simulink model "PV_Copy_of_Flight_controller_LQR_r2019a"  (R2019a)
settings: Solver=FixedStepDiscrete  StartTime=0.0  StopTime=10.0  FixedStep=sample_time  RelTol=1e-3
PreLoadFcn:
  | init_s
InitFcn:
  | init_s
undefined symbols (not defined in the file or in its folder): fw_params_fc, G, K, k1_nlin, k2_nlin, k3_nlin, mixer, sample_time
Description:
  | Template for Flight_controller.
  | This model should be used as a basis to develop a custom controller.
  | The controller can be deployed to the drone by means of the
  | ANT-X SLXtoPX4 tool for automatic controller code generation.
settings Model: Creator=flyart  LastModifiedBy=mariam
settings DataIOCC: ReturnWorkspaceOutputs=off
settings OptimizationCC: BlockReduction=off  DefaultParameterBehavior=Inlined  DefaultUnderspecifiedDataType=single  InlineInvariantSignals=on  EnhancedBackFolding=on  CachingGlobalReferences=on  LocalBlockOutputs=off
settings DebuggingCC: ParameterTunabilityLossMsg=error  ArithmeticOperatorsInVariantConditions=warning
settings HardwareCC: ProdBitPerPointer=32  ProdBitPerSizeT=32  ProdBitPerPtrDiffT=32  ProdLargestAtomicInteger=Long  ProdLargestAtomicFloat=Double  ProdWordSize=32  ProdHWDeviceType=ARM Compatible->ARM Cortex
settings SFSimCC: SimUseLocalCustomCode=off  MATLABDynamicMemAlloc=off
settings RTWCC: SystemTargetFile=ert.tlc  GenCodeOnly=on  TemplateMakefile=ert_default_tmf  GenerateReport=on  RTWUseLocalCustomCode=off  Toolchain=GNU gcc/g++ | gmake (64-bit Linux)  BuildConfiguration=Faster Runs  IncludeHyperlinkInReport=on  LaunchReport=on  TargetLang=C++  GenerateTraceInfo=on  GenerateTraceReport=on  GenerateTraceReportSl=on  GenerateTraceReportSf=on  GenerateTraceReportEml=on  GenerateCodeMetricsReport=on
settings CodeAppCC: ForceParamTrailComments=on  OperatorAnnotations=on  SimulinkDataObjDesc=on  SFDataObjDesc=on  MATLABFcnDesc=on  CustomSymbolStrGlobalVar=rt$N$M  CustomSymbolStrType=$N$M  InsertBlockDesc=on  StateflowObjectComments=on  MATLABSourceComments=on
settings ERTTargetCC: MultiwordLength=2048  MultiInstanceERTCode=on  CodeInterfacePackaging=C++ class  SupportNonFinite=off  SupportComplex=off  InlinedParameterPlacement=NonHierarchical  RootIOFormat=Structure reference  ERTCustomFileTemplate=example_file_process.tlc  ERTFilePackagingFormat=Compact

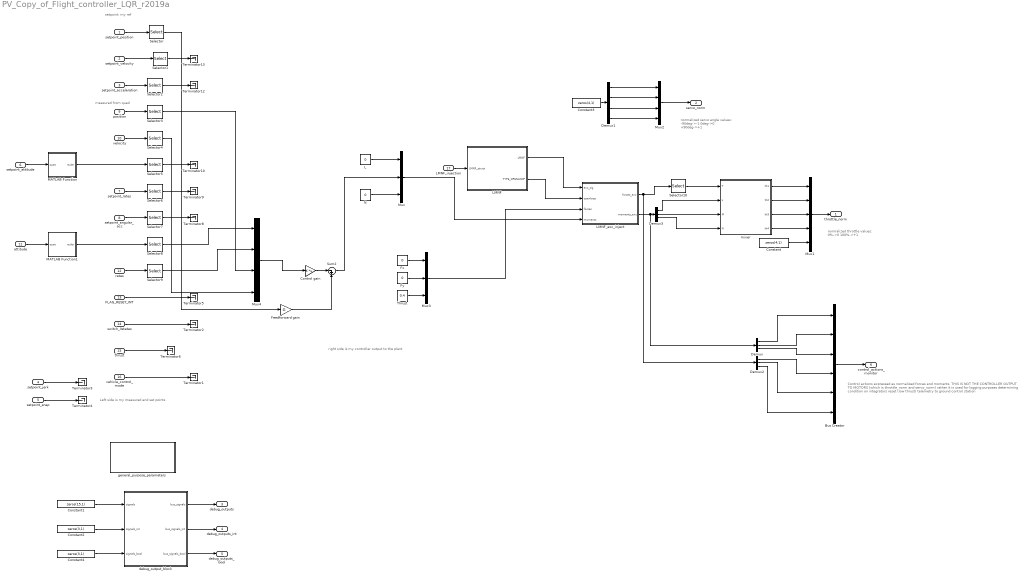
== system PV_Copy_of_Flight_controller_LQR_r2019a ==
  note: right side is my controller output to the plant
  note: Left side is my measured and set points
  note: measured from quad
  note: setpoint: my ref
  note: Control actions expressed as normalized forces and moments.
      | THIS IS NOT THE CONTROLLER OUTPUT TO MOTORS (which is throttle_norm and servo_norm)
      | rather it is used for
      | logging purposes
      | determining condition on integrators reset (low thrust)
      | telemetry to ground control station
  note: normalized servo angle values:
      | -90deg->-1
      | 0deg->0
      | +90deg->+1
  note: normalized throttle values:
      | 0%->0
      | 100%->+1
  setpoint_position : Inport  OutDataTypeStr=double  PortDimensions=3  SampleTime=sample_time
  setpoint_velocity : Inport  Port=2  OutDataTypeStr=double  PortDimensions=3  SampleTime=sample_time
  setpoint_acceleration : Inport  Port=3  OutDataTypeStr=double  PortDimensions=3  SampleTime=sample_time
  setpoint_jerk : Inport  Port=4  OutDataTypeStr=double  PortDimensions=3  SampleTime=sample_time
  setpoint_snap : Inport  Port=5  OutDataTypeStr=double  PortDimensions=3  SampleTime=sample_time
  setpoint_attitude : Inport  Port=6  OutDataTypeStr=double  PortDimensions=4  SampleTime=sample_time
  setpoint_rates : Inport  Port=7  OutDataTypeStr=double  Unit=rad/s  PortDimensions=3  SampleTime=sample_time
  setpoint_angular_acc : Inport  Port=8  OutDataTypeStr=double  Unit=rad/s^2  PortDimensions=3  SampleTime=sample_time
  position : Inport  Port=9  OutDataTypeStr=double  PortDimensions=3  SampleTime=sample_time
  velocity : Inport  Port=10  OutDataTypeStr=double  PortDimensions=3  SampleTime=sample_time
  attitude : Inport  Port=11  OutDataTypeStr=double  PortDimensions=4  SampleTime=sample_time
  rates : Inport  Port=12  OutDataTypeStr=double  Unit=rad/s  PortDimensions=3  SampleTime=sample_time
  FLAG_RESET_INT : Inport  Port=13  OutDataTypeStr=boolean  PortDimensions=1  SampleTime=sample_time
  switch_3states : Inport  Port=14  OutDataTypeStr=int8  PortDimensions=1  SampleTime=sample_time
  thrust : Inport  Port=15  OutDataTypeStr=double  PortDimensions=1  SampleTime=sample_time
  vehicle_control_mode : Inport  Port=16  OutDataTypeStr=Bus: vehicle_control_mode_bus  SampleTime=sample_time  BusOutputAsStruct=on
  LMNF_injection : Inport  Port=17  OutDataTypeStr=Bus: LMNF_injection_bus  SampleTime=sample_time  BusOutputAsStruct=on
  Bus Creator : BusCreator  Inputs=6  OutDataTypeStr=Bus: control_actions_bus  NonVirtualBus=on
      settings: InheritFromInputs=off
  Constant : Constant  Value=zeros(4,1)
  Constant1 : Constant  Value=zeros(15,1)  OutDataTypeStr=double
  Constant2 : Constant  Value=zeros(3,1)  OutDataTypeStr=int8
  Constant3 : Constant  Value=zeros(4,1)
  Constant4 : Constant  Value=zeros(3,1)  OutDataTypeStr=boolean
  Control gain : Gain  Gain=K  Multiplication=Matrix(K*u)
  Demux : Demux  Outputs=3
  Demux1 : Demux
  Demux2 : Demux  Outputs=3
  Demux3 : Demux  Outputs=3
  Feedforward gain : Gain  Gain=G
  Fx : Constant  Value=0
  Fy : Constant  Value=0
  L : Constant  Value=0
  LMNF : Subsystem
  LMNF_exc_inject : Subsystem
  MATLAB Function : MATLAB Function  TreatAsAtomicUnit=on
  MATLAB Function1 : MATLAB Function  TreatAsAtomicUnit=on
  Mux : Mux  Inputs=3
  Mux1 : Mux  Inputs=5
  Mux2 : Mux
  Mux3 : Mux  Inputs=3
  Mux4 : Mux
  N : Constant  Value=0
  Selector{,1..4} (5 alike) : Selector  InputPortWidth=3  IndexOptions=Index vector (dialog)  Indices=[1]  OutputSizes=1
  Selector10 : Selector  InputPortWidth=3  IndexOptions=Index vector (dialog)  Indices=[3]  OutputSizes=1
  Selector{5..9} (5 alike) : Selector  InputPortWidth=3  IndexOptions=Index vector (dialog)  Indices=[2]  OutputSizes=1
  Sum2 : Sum  Inputs=|-+
  Terminator{1..6,8..10,12..13} (11 alike) : Terminator
  Thrust : Constant  Value=0.4
  debug_output_block : Subsystem
  general_purpose_parameters : Subsystem
  mixer : Subsystem
  throttle_norm : Outport  OutDataTypeStr=double  PortDimensions=8  SampleTime=sample_time  VectorParamsAs1DForOutWhenUnconnected=on
  servo_norm : Outport  Port=2  OutDataTypeStr=double  PortDimensions=4  SampleTime=sample_time  VectorParamsAs1DForOutWhenUnconnected=on
  debug_outputs : Outport  Port=3  OutDataTypeStr=double  PortDimensions=15  SampleTime=sample_time  VectorParamsAs1DForOutWhenUnconnected=on
  debug_outputs_int : Outport  Port=4  OutDataTypeStr=int8  PortDimensions=3  SampleTime=sample_time  VectorParamsAs1DForOutWhenUnconnected=on
  debug_outputs_bool : Outport  Port=5  OutDataTypeStr=boolean  PortDimensions=3  SampleTime=sample_time  VectorParamsAs1DForOutWhenUnconnected=on
  control_actions_monitor : Outport  Port=6  OutDataTypeStr=Bus: control_actions_bus  SampleTime=sample_time  VectorParamsAs1DForOutWhenUnconnected=on
  wires:
  setpoint_acceleration/1 -> Selector2/1
  Selector2/1 -> Terminator12/1
  Mux/1 -> LMNF_exc_inject/4(moments)
  position/1 -> Selector3/1
  Constant2/1 -> debug_output_block/2(signals_int)
  Sum2/1 -> Mux/2
  FLAG_RESET_INT/1 -> Terminator5/1
  debug_output_block/3(bus_signals_bool) -> debug_outputs_bool/1
  Selector1/1 -> Terminator13/1
  Demux2/3 -> Bus Creator/6
  LMNF_exc_inject/2(moments_exc) -> Demux/1, Demux3/1
  LMNF/1(LMNF) -> LMNF_exc_inject/1(exc_sig)
  Constant4/1 -> debug_output_block/3(signals_bool)
  debug_output_block/1(bus_signals) -> debug_outputs/1
  Selector5/1 -> Terminator10/1
  Constant1/1 -> debug_output_block/1(signals)
  Demux2/2 -> Bus Creator/5
  LMNF_injection/1 -> LMNF/1(LMNF_struct)
  setpoint_attitude/1 -> MATLAB Function/1(quat)
  Demux3/2 -> mixer/3(M)
  LMNF_exc_inject/1(forces_exc) -> Demux2/1, Selector10/1
  Demux2/1 -> Bus Creator/4
  Fx/1 -> Mux3/1
  thrust/1 -> Terminator6/1
  Selector4/1 -> Mux4/4
  setpoint_velocity/1 -> Selector1/1
  Mux1/1 -> throttle_norm/1
  Demux/3 -> Bus Creator/3
  Constant/1 -> Mux1/5
  debug_output_block/2(bus_signals_int) -> debug_outputs_int/1
  switch_3states/1 -> Terminator2/1
  Demux3/3 -> mixer/4(N)
  rates/1 -> Selector9/1
  Demux3/1 -> mixer/2(L)
  MATLAB Function/1(euler) -> Selector5/1
  vehicle_control_mode/1 -> Terminator1/1
  Constant3/1 -> Demux1/1
  Demux/1 -> Bus Creator/1
  velocity/1 -> Selector4/1
  mixer/3(th3) -> Mux1/3
  setpoint_position/1 -> Selector/1
  setpoint_jerk/1 -> Terminator3/1
  attitude/1 -> MATLAB Function1/1(quat)
  Demux1/3 -> Mux2/3
  N/1 -> Mux/3
  Selector9/1 -> Mux4/2
  MATLAB Function1/1(euler) -> Selector8/1
  Bus Creator/1 -> control_actions_monitor/1
  Demux1/4 -> Mux2/4
  Demux1/2 -> Mux2/2
  mixer/1(th1) -> Mux1/1
  L/1 -> Mux/1
  Demux1/1 -> Mux2/1
  Selector10/1 -> mixer/1(T)
  LMNF/2(TYPE_OPENLOOP) -> LMNF_exc_inject/2(openloop)
  setpoint_angular_acc/1 -> Selector7/1
  Selector6/1 -> Terminator9/1
  Mux3/1 -> LMNF_exc_inject/3(forces)
  Fy/1 -> Mux3/2
  Selector7/1 -> Terminator8/1
  Selector3/1 -> Mux4/3
  setpoint_rates/1 -> Selector6/1
  setpoint_snap/1 -> Terminator4/1
  Demux/2 -> Bus Creator/2
  mixer/4(th4) -> Mux1/4
  mixer/2(th2) -> Mux1/2
  Mux2/1 -> servo_norm/1
  Selector8/1 -> Mux4/1
  Mux4/1 -> Control gain/1
  Control gain/1 -> Sum2/1
  Feedforward gain/1 -> Sum2/2
  Selector/1 -> Feedforward gain/1
  Thrust/1 -> Mux3/3

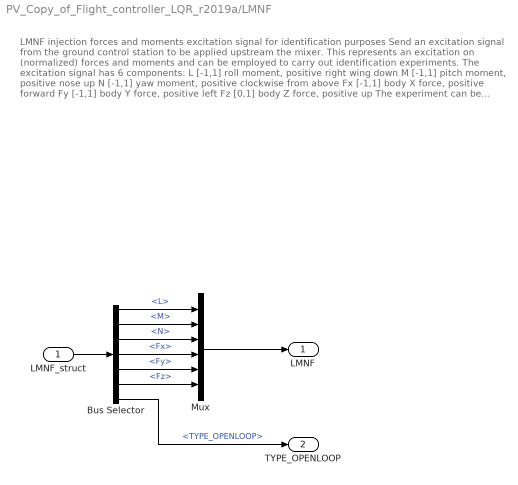
== system PV_Copy_of_Flight_controller_LQR_r2019a/LMNF ==
  note: LMNF injection
      | forces and moments excitation signal for identification purposes
      | Send an excitation signal from the ground control station to be applied upstream the mixer.
      | This represents an excitation on (normalized) forces and moments and can be employed
      | to carry out identification experiments.
      | The excitation signal has 6 components:
      | L [-1,1] roll moment, positive right wing down
      | M [-1,1] pitch moment, positive nose up
      | N [-1,1] yaw moment, positive clockwise from above
      | Fx [-1,1] body X force, positive forward
      | Fy [-1,1] body Y force, positive left
      | Fz [0,1] body Z force, positive up
      |
      | The experiment can be applied in open-loop or closed-loop (see the TYPE_OPENLOOP field).
      |
      | The number of applicable excitation components depends on the UAV configuration (namely, on the mixer)
      | e.g. a standard quadrotor configuration accepts roll/pitch/yaw/thrust as an input to the mixer, hence
      | the Fx and Fy components cannot be used; on the other hand, over-actuated architetures allow to use all excitation components.
  LMNF_struct : Inport
  Bus Selector : BusSelector  OutputSignals=L,M,N,Fx,Fy,Fz,TYPE_OPENLOOP
  Mux : Mux  Inputs=6
  LMNF : Outport  VectorParamsAs1DForOutWhenUnconnected=on
  TYPE_OPENLOOP : Outport  Port=2  VectorParamsAs1DForOutWhenUnconnected=on
  wires:
  LMNF_struct/1 -> Bus Selector/1
  Bus Selector/1 -> Mux/1  "<L>"
  Bus Selector/2 -> Mux/2  "<M>"
  Bus Selector/3 -> Mux/3  "<N>"
  Bus Selector/4 -> Mux/4  "<Fx>"
  Bus Selector/5 -> Mux/5  "<Fy>"
  Bus Selector/6 -> Mux/6  "<Fz>"
  Mux/1 -> LMNF/1
  Bus Selector/7 -> TYPE_OPENLOOP/1  "<TYPE_OPENLOOP>"

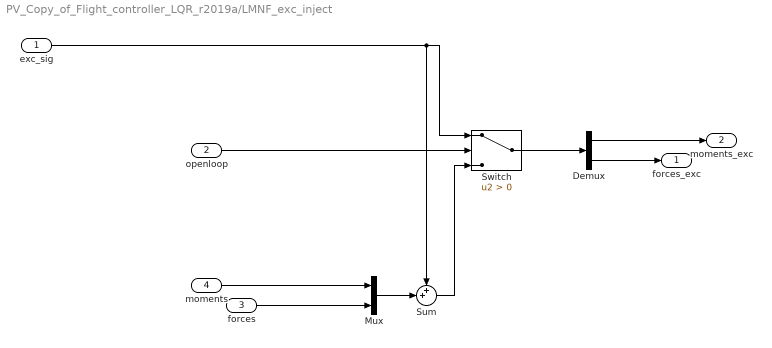
== system PV_Copy_of_Flight_controller_LQR_r2019a/LMNF_exc_inject ==
  exc_sig : Inport
  openloop : Inport  Port=2
  forces : Inport  Port=3
  moments : Inport  Port=4
  Demux : Demux  Outputs=2
  Mux : Mux  Inputs=2
  Sum : Sum  Inputs=++|
  Switch : Switch  Criteria=u2 > Threshold
  forces_exc : Outport  VectorParamsAs1DForOutWhenUnconnected=on
  moments_exc : Outport  Port=2  VectorParamsAs1DForOutWhenUnconnected=on
  wires:
  openloop/1 -> Switch/2
  Mux/1 -> Sum/2
  Switch/1 -> Demux/1
  Sum/1 -> Switch/3
  moments/1 -> Mux/1
  forces/1 -> Mux/2
  Demux/2 -> forces_exc/1
  Demux/1 -> moments_exc/1
  exc_sig/1 -> Sum/1, Switch/1

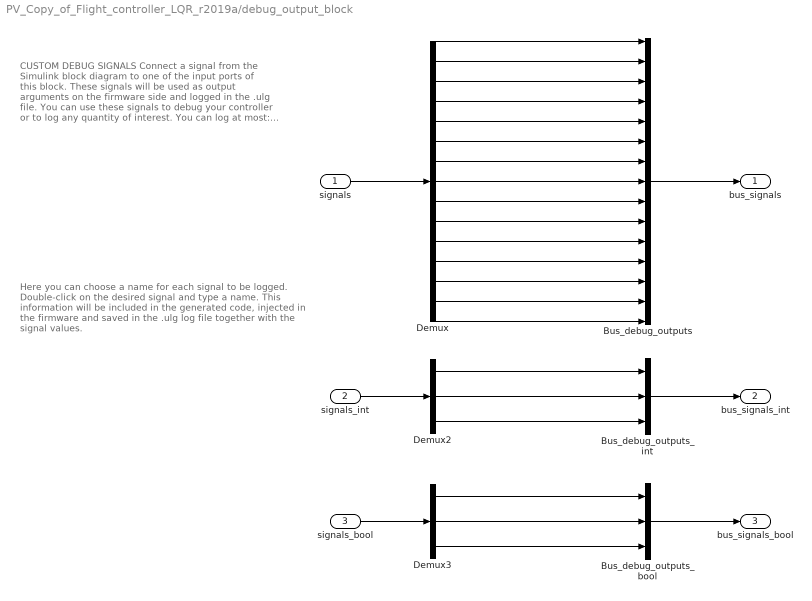
== system PV_Copy_of_Flight_controller_LQR_r2019a/debug_output_block ==
  note: CUSTOM DEBUG SIGNALS
      |
      | Connect a signal from the Simulink block diagram
      | to one of the input ports of this block.
      | These signals will be used as output arguments
      | on the firmware side and logged in the .ulg file.
      | You can use these signals to debug your controller
      | or to log any quantity of interest.
      |
      | You can log at most:
      | _ 15 signal of double type
      | _ 3 int
      | _ 3 bool
  note: Here you can choose a name for each signal to be logged.
      | Double-click on the desired signal and type a name.
      | This information will be included in the generated code,
      | injected in the firmware and saved in the .ulg log file
      | together with the signal values.
  signals : Inport
  signals_int : Inport  Port=2
  signals_bool : Inport  Port=3
  Bus_debug_outputs : BusCreator  Inputs=15
  Bus_debug_outputs_bool : BusCreator  Inputs=3
  Bus_debug_outputs_int : BusCreator  Inputs=3
  Demux : Demux  Outputs=15
  Demux2 : Demux  Outputs=3
  Demux3 : Demux  Outputs=3
  bus_signals : Outport  VectorParamsAs1DForOutWhenUnconnected=on
  bus_signals_int : Outport  Port=2  VectorParamsAs1DForOutWhenUnconnected=on
  bus_signals_bool : Outport  Port=3  VectorParamsAs1DForOutWhenUnconnected=on
  wires:
  Bus_debug_outputs/1 -> bus_signals/1
  Demux/3 -> Bus_debug_outputs/3
  Demux/10 -> Bus_debug_outputs/10
  Demux/9 -> Bus_debug_outputs/9
  Demux/14 -> Bus_debug_outputs/14
  Demux/12 -> Bus_debug_outputs/12
  Demux/2 -> Bus_debug_outputs/2
  Demux/15 -> Bus_debug_outputs/15
  Demux/11 -> Bus_debug_outputs/11
  Demux/8 -> Bus_debug_outputs/8
  Demux/1 -> Bus_debug_outputs/1
  Demux/6 -> Bus_debug_outputs/6
  Demux/4 -> Bus_debug_outputs/4
  Demux/13 -> Bus_debug_outputs/13
  Demux/5 -> Bus_debug_outputs/5
  Demux/7 -> Bus_debug_outputs/7
  signals/1 -> Demux/1
  Demux2/3 -> Bus_debug_outputs_int/3
  Demux2/1 -> Bus_debug_outputs_int/1
  Demux2/2 -> Bus_debug_outputs_int/2
  Bus_debug_outputs_int/1 -> bus_signals_int/1
  signals_int/1 -> Demux2/1
  signals_bool/1 -> Demux3/1
  Demux3/1 -> Bus_debug_outputs_bool/1
  Demux3/2 -> Bus_debug_outputs_bool/2
  Demux3/3 -> Bus_debug_outputs_bool/3
  Bus_debug_outputs_bool/1 -> bus_signals_bool/1

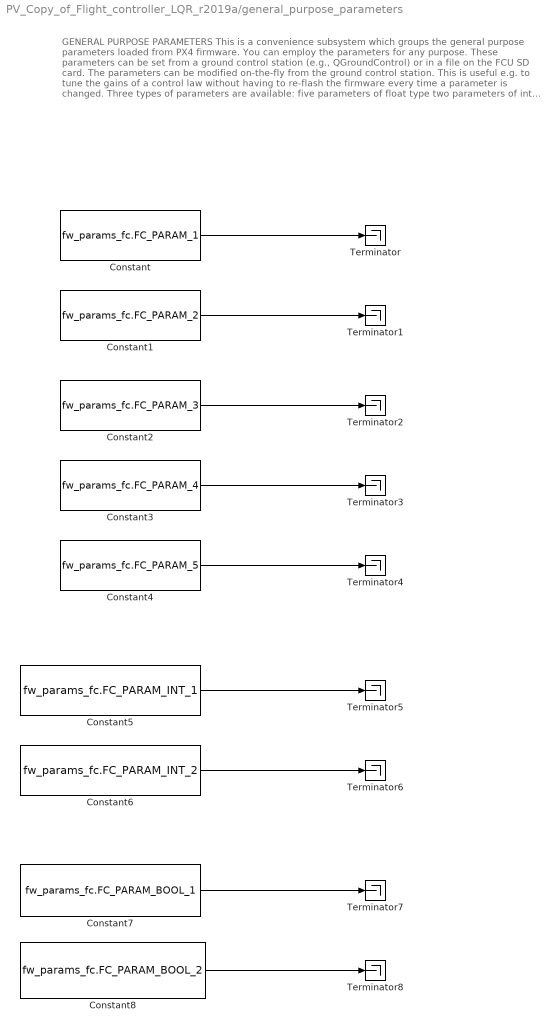
== system PV_Copy_of_Flight_controller_LQR_r2019a/general_purpose_parameters ==
  note: GENERAL PURPOSE PARAMETERS
      |
      | This is a convenience subsystem which groups the general purpose parameters loaded from PX4 firmware.
      | You can employ the parameters for any purpose.
      | These parameters can be set from a ground control station (e.g., QGroundControl) or in a file on the FCU SD card.
      | The parameters can be modified on-the-fly from the ground control station.
      | This is useful e.g. to tune the gains of a control law without having to re-flash the firmware every time a parameter is changed.
      |
      | Three types of parameters are available:
      | five parameters of float type
      | two parameters of int type
      | two parameters of bool type
  Constant : Constant  Value=fw_params_fc.FC_PARAM_1
  Constant1 : Constant  Value=fw_params_fc.FC_PARAM_2
  Constant2 : Constant  Value=fw_params_fc.FC_PARAM_3
  Constant3 : Constant  Value=fw_params_fc.FC_PARAM_4
  Constant4 : Constant  Value=fw_params_fc.FC_PARAM_5
  Constant5 : Constant  Value=fw_params_fc.FC_PARAM_INT_1
  Constant6 : Constant  Value=fw_params_fc.FC_PARAM_INT_2
  Constant7 : Constant  Value=fw_params_fc.FC_PARAM_BOOL_1
  Constant8 : Constant  Value=fw_params_fc.FC_PARAM_BOOL_2
  Terminator{,1..8} (9 alike) : Terminator
  wires:
  Constant/1 -> Terminator/1
  Constant1/1 -> Terminator1/1
  Constant2/1 -> Terminator2/1
  Constant3/1 -> Terminator3/1
  Constant4/1 -> Terminator4/1
  Constant5/1 -> Terminator5/1
  Constant6/1 -> Terminator6/1
  Constant7/1 -> Terminator7/1
  Constant8/1 -> Terminator8/1

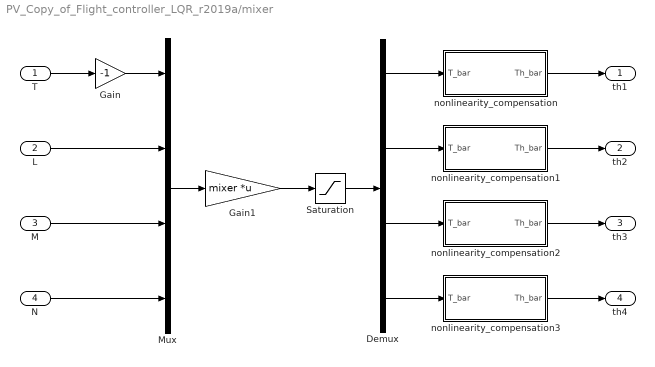
== system PV_Copy_of_Flight_controller_LQR_r2019a/mixer ==
  T : Inport
  L : Inport  Port=2
  M : Inport  Port=3
  N : Inport  Port=4
  Demux : Demux
  Gain : Gain  Gain=-1
  Gain1 : Gain  Gain=mixer  Multiplication=Matrix(K*u)
  Mux : Mux
  Saturation : Saturate  UpperLimit=1  LowerLimit=0
  nonlinearity_compensation : Subsystem
  nonlinearity_compensation1 : Subsystem
  nonlinearity_compensation2 : Subsystem
  nonlinearity_compensation3 : Subsystem
  th1 : Outport  VectorParamsAs1DForOutWhenUnconnected=on
  th2 : Outport  Port=2  VectorParamsAs1DForOutWhenUnconnected=on
  th3 : Outport  Port=3  VectorParamsAs1DForOutWhenUnconnected=on
  th4 : Outport  Port=4  VectorParamsAs1DForOutWhenUnconnected=on
  wires:
  T/1 -> Gain/1
  L/1 -> Mux/2
  M/1 -> Mux/3
  N/1 -> Mux/4
  nonlinearity_compensation/1(Th_bar) -> th1/1
  Gain/1 -> Mux/1
  Mux/1 -> Gain1/1
  Gain1/1 -> Saturation/1
  Demux/1 -> nonlinearity_compensation/1(T_bar)
  Saturation/1 -> Demux/1
  Demux/4 -> nonlinearity_compensation3/1(T_bar)
  nonlinearity_compensation3/1(Th_bar) -> th4/1
  Demux/3 -> nonlinearity_compensation2/1(T_bar)
  nonlinearity_compensation2/1(Th_bar) -> th3/1
  Demux/2 -> nonlinearity_compensation1/1(T_bar)
  nonlinearity_compensation1/1(Th_bar) -> th2/1

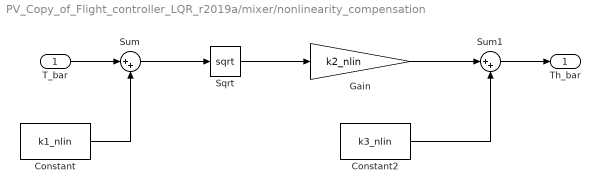
== system PV_Copy_of_Flight_controller_LQR_r2019a/mixer/nonlinearity_compensation ==
  T_bar : Inport
  Constant : Constant  Value=k1_nlin
  Constant2 : Constant  Value=k3_nlin
  Gain : Gain  Gain=k2_nlin
  Sqrt : Sqrt  SaturateOnIntegerOverflow=on
  Sum : Sum  Inputs=|++
  Sum1 : Sum  Inputs=|++
  Th_bar : Outport  VectorParamsAs1DForOutWhenUnconnected=on
  wires:
  T_bar/1 -> Sum/1
  Constant/1 -> Sum/2
  Sum/1 -> Sqrt/1
  Sqrt/1 -> Gain/1
  Constant2/1 -> Sum1/2
  Gain/1 -> Sum1/1
  Sum1/1 -> Th_bar/1

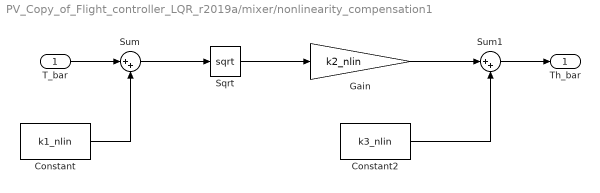
== system PV_Copy_of_Flight_controller_LQR_r2019a/mixer/nonlinearity_compensation1 ==
  T_bar : Inport
  Constant : Constant  Value=k1_nlin
  Constant2 : Constant  Value=k3_nlin
  Gain : Gain  Gain=k2_nlin
  Sqrt : Sqrt  SaturateOnIntegerOverflow=on
  Sum : Sum  Inputs=|++
  Sum1 : Sum  Inputs=|++
  Th_bar : Outport  VectorParamsAs1DForOutWhenUnconnected=on
  wires:
  T_bar/1 -> Sum/1
  Constant/1 -> Sum/2
  Sum/1 -> Sqrt/1
  Sqrt/1 -> Gain/1
  Constant2/1 -> Sum1/2
  Gain/1 -> Sum1/1
  Sum1/1 -> Th_bar/1

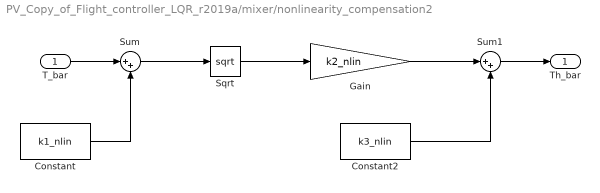
== system PV_Copy_of_Flight_controller_LQR_r2019a/mixer/nonlinearity_compensation2 ==
  T_bar : Inport
  Constant : Constant  Value=k1_nlin
  Constant2 : Constant  Value=k3_nlin
  Gain : Gain  Gain=k2_nlin
  Sqrt : Sqrt  SaturateOnIntegerOverflow=on
  Sum : Sum  Inputs=|++
  Sum1 : Sum  Inputs=|++
  Th_bar : Outport  VectorParamsAs1DForOutWhenUnconnected=on
  wires:
  T_bar/1 -> Sum/1
  Constant/1 -> Sum/2
  Sum/1 -> Sqrt/1
  Sqrt/1 -> Gain/1
  Constant2/1 -> Sum1/2
  Gain/1 -> Sum1/1
  Sum1/1 -> Th_bar/1

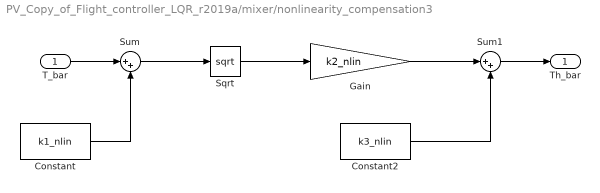
== system PV_Copy_of_Flight_controller_LQR_r2019a/mixer/nonlinearity_compensation3 ==
  T_bar : Inport
  Constant : Constant  Value=k1_nlin
  Constant2 : Constant  Value=k3_nlin
  Gain : Gain  Gain=k2_nlin
  Sqrt : Sqrt  SaturateOnIntegerOverflow=on
  Sum : Sum  Inputs=|++
  Sum1 : Sum  Inputs=|++
  Th_bar : Outport  VectorParamsAs1DForOutWhenUnconnected=on
  wires:
  T_bar/1 -> Sum/1
  Constant/1 -> Sum/2
  Sum/1 -> Sqrt/1
  Sqrt/1 -> Gain/1
  Constant2/1 -> Sum1/2
  Gain/1 -> Sum1/1
  Sum1/1 -> Th_bar/1

== matlab function PV_Copy_of_Flight_controller_LQR_r2019a/MATLAB Function1 ==
  data: quat input; euler output
function euler = quatToEuler( quat )
%	Converts a quaternion vector to ZYX Euler angles (RPY)
%
%   euler = quatToEuler( quat )
%
%   The quaternion (quat) must be written as a 4-by-1 matrix with the scalar
%   element as the fourth component.
%   The returned Euler angles vector will be written in radiants as a 3-by-1 vector.
%
%   References:
%	[1] Markley, F. Landis. "Attitude error representations for Kalman filtering." 
%       Journal of guidance control and dynamics 26.2 (2003): 311-317.

norm = sqrt(quat(1)^2 + quat(2)^2 + quat(3)^2 + quat(4)^2);
quat(1) = quat(1) / norm;
quat(2) = quat(2) / norm;
quat(3) = quat(3) / norm;
quat(4) = quat(4) / norm;

A11 = quat(1)^2 - quat(2)^2 - quat(3)^2 + quat(4)^2;
A12 = 2*quat(1)*quat(2) + 2*quat(3)*quat(4);
A13 = 2*quat(1)*quat(3) - 2*quat(2)*quat(4);
A23 = 2*quat(1)*quat(4) + 2*quat(2)*quat(3);
A33 = - quat(1)^2 - quat(2)^2 + quat(3)^2 + quat(4)^2;

phi = atan2(A23, A33);
theta = - asin(A13);
psi = atan2(A12, A11);

euler = [ phi, theta, psi]';

end

== matlab function PV_Copy_of_Flight_controller_LQR_r2019a/MATLAB Function ==
  data: quat input; euler output
function euler = quatToEuler( quat )
%	Converts a quaternion vector to ZYX Euler angles (RPY)
%
%   euler = quatToEuler( quat )
%
%   The quaternion (quat) must be written as a 4-by-1 matrix with the scalar
%   element as the fourth component.
%   The returned Euler angles vector will be written in radiants as a 3-by-1 vector.
%
%   References:
%	[1] Markley, F. Landis. "Attitude error representations for Kalman filtering." 
%       Journal of guidance control and dynamics 26.2 (2003): 311-317.

norm = sqrt(quat(1)^2 + quat(2)^2 + quat(3)^2 + quat(4)^2);
quat(1) = quat(1) / norm;
quat(2) = quat(2) / norm;
quat(3) = quat(3) / norm;
quat(4) = quat(4) / norm;

A11 = quat(1)^2 - quat(2)^2 - quat(3)^2 + quat(4)^2;
A12 = 2*quat(1)*quat(2) + 2*quat(3)*quat(4);
A13 = 2*quat(1)*quat(3) - 2*quat(2)*quat(4);
A23 = 2*quat(1)*quat(4) + 2*quat(2)*quat(3);
A33 = - quat(1)^2 - quat(2)^2 + quat(3)^2 + quat(4)^2;

phi = atan2(A23, A33);
theta = - asin(A13);
psi = atan2(A12, A11);

euler = [ phi, theta, psi]';

end
